simulink model "one_loop_dcmotor"  (R2022a)
settings: Solver=VariableStepAuto  StartTime=0.0  StopTime=10  MaxStep=1e-5  RelTol=1e-3
values from neighbouring files (symbols this model uses):
  Ce = 0.131    [params.m]
  Ra = 1.5    [params.m]
  TL = 0.0144    [params.m]
  Tm = 0.18    [params.m]
libraries: spsDCVoltageSourceLib x3, spsUniversalBridgeLib x3, simulink x3, spsVoltageMeasurementLib x3, spsMeanLib x2, spspowerguiLib x1
settings Model: Creator=lzd  LastModifiedBy=lzd

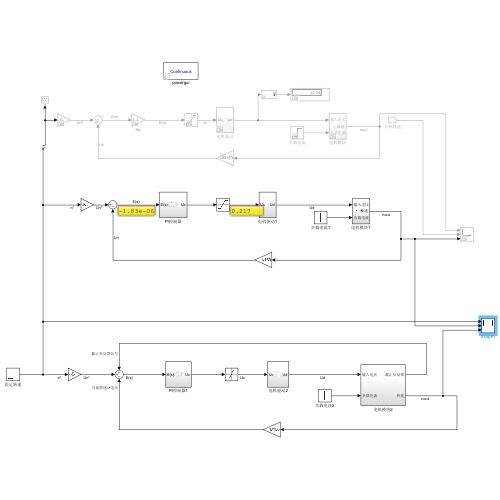
[thumbnail: Simulink's stored preview of the top-level diagram]
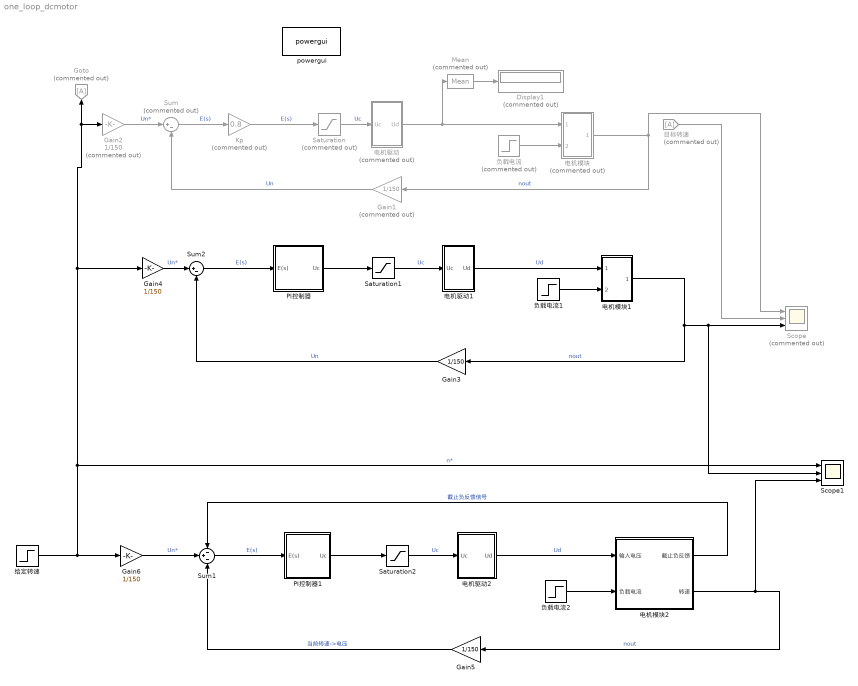
== system one_loop_dcmotor ==
  Display1 : Display  Commented=on
  Gain1 : Gain  Commented=on  Gain=1/150
  Gain2 : Gain  Commented=on  Gain=1/150
  Gain{3..6} (4 alike) : Gain  Gain=1/150
  Goto : Goto  Commented=on
  Kp : Gain  Commented=on  Gain=0.8
  Mean : spsMeanLib/Mean  Commented=on  Freq=60  Vinit=0  Ts=0
  PI控制器 : Subsystem
  PI控制器1 : Subsystem
  Saturation : Saturate  Commented=on  UpperLimit=5  LowerLimit=-5
  Saturation1 : Saturate  UpperLimit=5  LowerLimit=-5
  Saturation2 : Saturate  UpperLimit=5  LowerLimit=-5
  Scope : Scope  Commented=on  NumInputPorts=3
  Scope1 : Scope  NumInputPorts=3
  Sum : Sum  Commented=on  Inputs=|+-
  Sum1 : Sum  Inputs=-+-
  Sum2 : Sum  Inputs=|+-
  powergui : spspowerguiLib/powergui  Priority=1  SimulationMode=Continuous  SampleTime=50e-6  frequency=60  Iterations=50  frequencyindice=0  Pbase=100e6  ErrMax=1e-4  UnitsV=kV  UnitsW=MW  buscounter=0  FunctionMessages=off  echomessages=off  EnableUseOfTLC=off  CurrentSourceSwitches=off  DisableSnubberDevices=off  DisableRonSwitches=off  DisableVfSwitches=off  DisplayEquations=off  AutomaticDiscreteSolvers=off  SolverType=Tustin/Backward Euler (TBE)  Interpol=off  ExternalGateDelay=off  methode=off  Ts=100  x0status=blocks  SPID=on  SwTol=0  HookPort=off  NonlinearTolerance=1e-4  nMaxIteration=100  ContinueOnMaxIteration=off  RestoreLinks=warning  ResistiveCurrentMeasurement=off  Frange=[0:2:500]  Ylog=off  Xlog=on  ShowGrid=off  save=off  variable=ZData  structure=0  ZoomFFT=off  StartTime=0.0  cycles=1  DisplayStyle=1  fundamental=60  FreqAxis=off  MaxFrequency=1000  frequencyindicesteady=1  RmsSteady=1  display=off
  电机模块 : Subsystem  Commented=on
  电机模块1 : Subsystem
  电机模块2 : Subsystem
  电机驱动 : Subsystem  Commented=on
  电机驱动1 : Subsystem
  电机驱动2 : Subsystem
  目标转速 : From  Commented=on
  给定转速 : Step  Time=0.02  After=1300  SampleTime=0
  负载电流 : Step  Commented=on  Time=0.1  After=15.6  SampleTime=0
  负载电流1 : Step  Time=0.1  After=15.6  SampleTime=0
  负载电流2 : Step  Time=0.1  After=15.6  SampleTime=0
  wires:
  Mean/1 -> Display1/1
  电机模块/1(转速) -> Scope/1, Gain1/1  "nout"
  负载电流/1 -> 电机模块/2(负载电流)
  Sum/1 -> Kp/1  "E(s)"
  Gain1/1 -> Sum/2  "Un"
  Gain2/1 -> Sum/1  "Un*"
  电机驱动/1(Ud) -> 电机模块/1(输入电压), Mean/1
  Saturation/1 -> 电机驱动/1(Uc)  "Uc"
  目标转速/1 -> Scope/2
  Kp/1 -> Saturation/1  "E(s)"
  Saturation1/1 -> 电机驱动1/1(Uc)  "Uc"
  电机驱动1/1(Ud) -> 电机模块1/1(输入电压)  "Ud"
  Gain4/1 -> Sum2/1  "Un*"
  Gain3/1 -> Sum2/2  "Un"
  负载电流1/1 -> 电机模块1/2(负载电流)
  电机模块1/1(转速) -> Gain3/1, Scope1/2, Scope/3  "nout"
  Sum2/1 -> PI控制器/1(E(s))  "E(s)"
  PI控制器/1(Uc) -> Saturation1/1
  PI控制器1/1(Uc) -> Saturation2/1
  电机模块2/2(转速) -> Scope1/3, Gain5/1  "nout"
  负载电流2/1 -> 电机模块2/2(负载电流)
  给定转速/1 -> Scope1/1, Gain2/1, Goto/1, Gain4/1, Gain6/1  "n*"
  电机驱动2/1(Ud) -> 电机模块2/1(输入电压)  "Ud"
  Saturation2/1 -> 电机驱动2/1(Uc)  "Uc"
  Sum1/1 -> PI控制器1/1(E(s))  "E(s)"
  Gain6/1 -> Sum1/2  "Un*"
  电机模块2/1(截止负反馈) -> Sum1/1  "截止负反馈信号"
  Gain5/1 -> Sum1/3  "当前转速->电压"

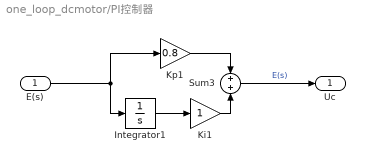
== system one_loop_dcmotor/PI控制器 ==
  E(s) : Inport
  Integrator1 : Integrator  LimitOutput=on  UpperSaturationLimit=5  LowerSaturationLimit=-5
  Ki1 : Gain
  Kp1 : Gain  Gain=0.8
  Sum3 : Sum  Inputs=+|+
  Uc : Outport
  wires:
  E(s)/1 -> Integrator1/1, Kp1/1
  Ki1/1 -> Sum3/2
  Integrator1/1 -> Ki1/1
  Kp1/1 -> Sum3/1
  Sum3/1 -> Uc/1  "E(s)"

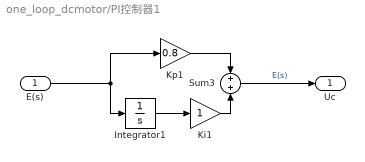
== system one_loop_dcmotor/PI控制器1 ==
  E(s) : Inport
  Integrator1 : Integrator  LimitOutput=on  UpperSaturationLimit=5  LowerSaturationLimit=-5
  Ki1 : Gain
  Kp1 : Gain  Gain=0.8
  Sum3 : Sum  Inputs=+|+
  Uc : Outport
  wires:
  Sum3/1 -> Uc/1  "E(s)"
  Kp1/1 -> Sum3/1
  Integrator1/1 -> Ki1/1
  Ki1/1 -> Sum3/2
  E(s)/1 -> Kp1/1, Integrator1/1

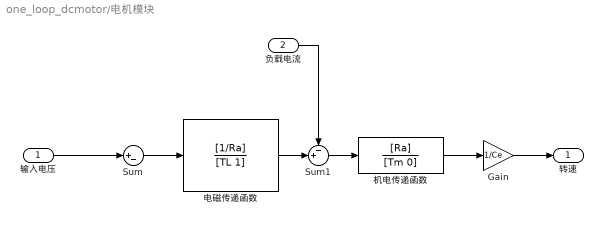
== system one_loop_dcmotor/电机模块 ==
  输入电压 : Inport
  负载电流 : Inport  Port=2
  Gain : Gain  Gain=1/Ce
  Sum : Sum  Inputs=|+-
  Sum1 : Sum  Inputs=-+|
  机电传递函数 : TransferFcn  Numerator=[Ra]  Denominator=[Tm 0]
  电磁传递函数 : TransferFcn  Numerator=[1/Ra]  Denominator=[TL 1]
  转速 : Outport
  wires:
  输入电压/1 -> Sum/1
  电磁传递函数/1 -> Sum1/2
  负载电流/1 -> Sum1/1
  Sum1/1 -> 机电传递函数/1
  机电传递函数/1 -> Gain/1
  Sum/1 -> 电磁传递函数/1
  Gain/1 -> 转速/1

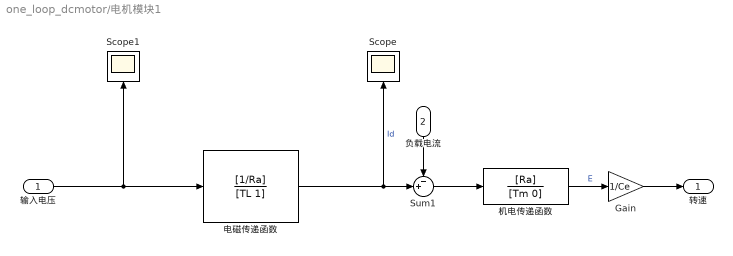
== system one_loop_dcmotor/电机模块1 ==
  输入电压 : Inport
  负载电流 : Inport  Port=2
  Gain : Gain  Gain=1/Ce
  Scope : Scope
  Scope1 : Scope
  Sum1 : Sum  Inputs=-+|
  机电传递函数 : TransferFcn  Numerator=[Ra]  Denominator=[Tm 0]
  电磁传递函数 : TransferFcn  Numerator=[1/Ra]  Denominator=[TL 1]
  转速 : Outport
  wires:
  Gain/1 -> 转速/1
  输入电压/1 -> 电磁传递函数/1, Scope1/1
  机电传递函数/1 -> Gain/1  "E"
  Sum1/1 -> 机电传递函数/1
  负载电流/1 -> Sum1/1
  电磁传递函数/1 -> Sum1/2, Scope/1  "Id"

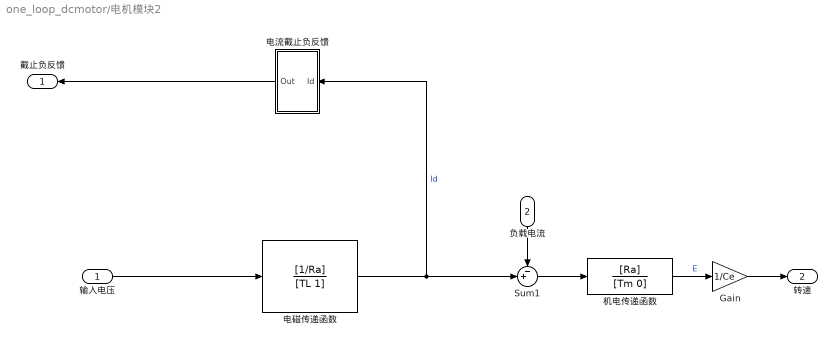
== system one_loop_dcmotor/电机模块2 ==
  输入电压 : Inport
  负载电流 : Inport  Port=2
  Gain : Gain  Gain=1/Ce
  Sum1 : Sum  Inputs=-+|
  机电传递函数 : TransferFcn  Numerator=[Ra]  Denominator=[Tm 0]
  电流截止负反馈 : Subsystem
  电磁传递函数 : TransferFcn  Numerator=[1/Ra]  Denominator=[TL 1]
  截止负反馈 : Outport
  转速 : Outport  Port=2
  wires:
  电磁传递函数/1 -> Sum1/2, 电流截止负反馈/1(Id)  "Id"
  负载电流/1 -> Sum1/1
  Sum1/1 -> 机电传递函数/1
  机电传递函数/1 -> Gain/1  "E"
  输入电压/1 -> 电磁传递函数/1
  Gain/1 -> 转速/1
  电流截止负反馈/1(Out) -> 截止负反馈/1

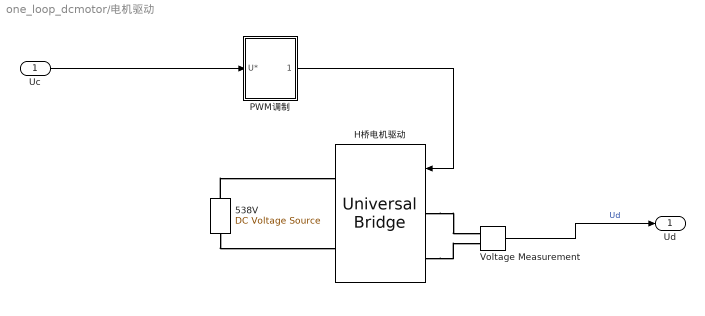
== system one_loop_dcmotor/电机驱动 ==
  Uc : Inport
  538V : spsDCVoltageSourceLib/DC Voltage Source  Amplitude=538  Measurements=None
  H桥电机驱动 : spsUniversalBridgeLib/Universal Bridge  Arms=2  SnubberResistance=1e5  SnubberCapacitance=inf  Device=MOSFET / Diodes  Ron=1e-3  Lon=0  ForwardVoltages="[  0  0  ]"  ForwardVoltage=0  GTOparameters=[ 10e-6 , 20e-6 ]  IGBTparameters=[ 1e-6 , 2e-6 ]  Measurements=None  Measurements_2=None  converterType=Rectifier
  PWM调制 : Subsystem
  Voltage Measurement : spsVoltageMeasurementLib/Voltage Measurement  PhasorSimulation=off  OutputType=Complex  PSBequivalent=0
  Ud : Outport
  wires:
  Voltage Measurement/1 -> Ud/1  "Ud"
  PWM调制/1(4*PWM) -> H桥电机驱动/1
  Uc/1 -> PWM调制/1(U*)
  connections:
  H桥电机驱动/LConn2 -- Voltage Measurement/LConn2
  538V/LConn1 -- H桥电机驱动/RConn2
  538V/RConn1 -- H桥电机驱动/RConn1
  H桥电机驱动/LConn1 -- Voltage Measurement/LConn1

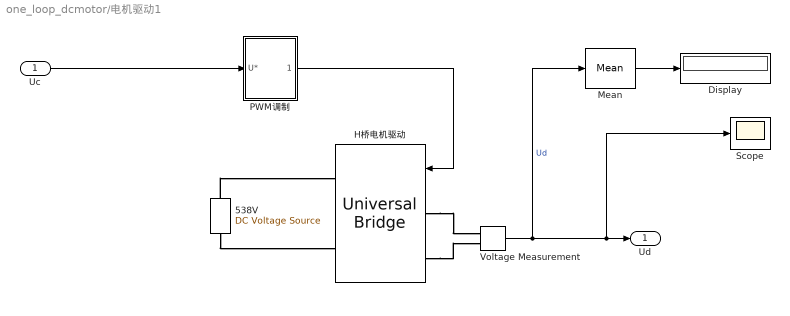
== system one_loop_dcmotor/电机驱动1 ==
  Uc : Inport
  538V : spsDCVoltageSourceLib/DC Voltage Source  Amplitude=538  Measurements=None
  Display : Display
  H桥电机驱动 : spsUniversalBridgeLib/Universal Bridge  Arms=2  SnubberResistance=1e5  SnubberCapacitance=inf  Device=MOSFET / Diodes  Ron=1e-3  Lon=0  ForwardVoltages="[  0  0  ]"  ForwardVoltage=0  GTOparameters=[ 10e-6 , 20e-6 ]  IGBTparameters=[ 1e-6 , 2e-6 ]  Measurements=None  Measurements_2=None  converterType=Rectifier
  Mean : spsMeanLib/Mean  Freq=50  Vinit=0  Ts=0
  PWM调制 : Subsystem
  Scope : Scope
  Voltage Measurement : spsVoltageMeasurementLib/Voltage Measurement  PhasorSimulation=off  OutputType=Complex  PSBequivalent=0
  Ud : Outport
  wires:
  Uc/1 -> PWM调制/1(U*)
  PWM调制/1(4*PWM) -> H桥电机驱动/1
  Voltage Measurement/1 -> Mean/1, Scope/1, Ud/1  "Ud"
  Mean/1 -> Display/1
  connections:
  H桥电机驱动/LConn1 -- Voltage Measurement/LConn1
  538V/RConn1 -- H桥电机驱动/RConn1
  538V/LConn1 -- H桥电机驱动/RConn2
  H桥电机驱动/LConn2 -- Voltage Measurement/LConn2

== system one_loop_dcmotor/电机驱动2 ==
  Uc : Inport
  538V : spsDCVoltageSourceLib/DC Voltage Source  Amplitude=538  Measurements=None
  H桥电机驱动 : spsUniversalBridgeLib/Universal Bridge  Arms=2  SnubberResistance=1e5  SnubberCapacitance=inf  Device=MOSFET / Diodes  Ron=1e-3  Lon=0  ForwardVoltages="[  0  0  ]"  ForwardVoltage=0  GTOparameters=[ 10e-6 , 20e-6 ]  IGBTparameters=[ 1e-6 , 2e-6 ]  Measurements=None  Measurements_2=None  converterType=Rectifier
  PWM调制 : Subsystem
  Voltage Measurement : spsVoltageMeasurementLib/Voltage Measurement  PhasorSimulation=off  OutputType=Complex  PSBequivalent=0
  Ud : Outport
  wires:
  Voltage Measurement/1 -> Ud/1  "Ud"
  PWM调制/1(4*PWM) -> H桥电机驱动/1
  Uc/1 -> PWM调制/1(U*)
  connections:
  H桥电机驱动/LConn2 -- Voltage Measurement/LConn2
  538V/LConn1 -- H桥电机驱动/RConn2
  538V/RConn1 -- H桥电机驱动/RConn1
  H桥电机驱动/LConn1 -- Voltage Measurement/LConn1

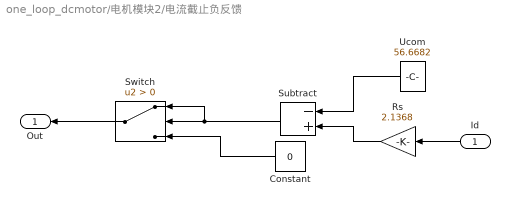
== system one_loop_dcmotor/电机模块2/电流截止负反馈 ==
  Id : Inport
  Constant : Constant  Value=0
  Rs : Gain  Gain=2.1368
  Subtract : Sum  Inputs=-+
  Switch : Switch  Criteria=u2 > Threshold  SaturateOnIntegerOverflow=off  InputSameDT=off
  Ucom : Constant  Value=56.6682
  Out : Outport
  wires:
  Subtract/1 -> Switch/2, Switch/1
  Id/1 -> Rs/1
  Rs/1 -> Subtract/2
  Constant/1 -> Switch/3
  Ucom/1 -> Subtract/1
  Switch/1 -> Out/1

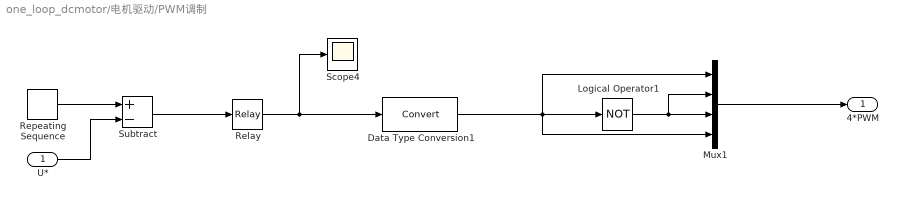
== system one_loop_dcmotor/电机驱动/PWM调制 ==
  U* : Inport
  Data Type Conversion1 : DataTypeConversion  SaturateOnIntegerOverflow=off  RndMeth=Floor
  Logical Operator1 : Logic  Operator=NOT  AllPortsSameDT=off  OutDataTypeStr=boolean
  Mux1 : Mux
  Relay : Relay  OnOutputValue=0  OffOutputValue=1
  Repeating Sequence : simulink/Sources/Repeating Sequence  rep_seq_t=[0 1/8000]  rep_seq_y=[-5 +5]
  Scope4 : Scope
  Subtract : Sum  Inputs=+-
  4*PWM : Outport
  wires:
  Relay/1 -> Scope4/1, Data Type Conversion1/1
  Data Type Conversion1/1 -> Mux1/4, Mux1/1, Logical Operator1/1
  Subtract/1 -> Relay/1
  Logical Operator1/1 -> Mux1/2, Mux1/3
  Repeating Sequence/1 -> Subtract/1
  Mux1/1 -> 4*PWM/1
  U*/1 -> Subtract/2

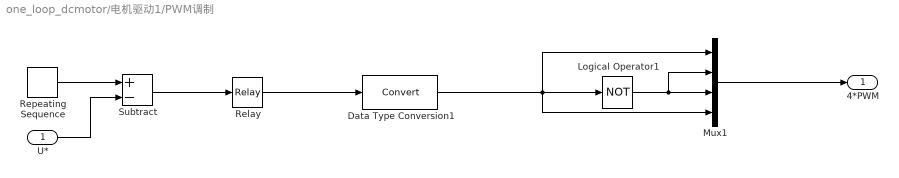
== system one_loop_dcmotor/电机驱动1/PWM调制 ==
  U* : Inport
  Data Type Conversion1 : DataTypeConversion  SaturateOnIntegerOverflow=off  RndMeth=Floor
  Logical Operator1 : Logic  Operator=NOT  AllPortsSameDT=off  OutDataTypeStr=boolean
  Mux1 : Mux
  Relay : Relay  OnOutputValue=0  OffOutputValue=1
  Repeating Sequence : simulink/Sources/Repeating Sequence  rep_seq_t=[0 1/8000]  rep_seq_y=[-5 +5]
  Subtract : Sum  Inputs=+-
  4*PWM : Outport
  wires:
  U*/1 -> Subtract/2
  Mux1/1 -> 4*PWM/1
  Repeating Sequence/1 -> Subtract/1
  Logical Operator1/1 -> Mux1/3, Mux1/2
  Subtract/1 -> Relay/1
  Data Type Conversion1/1 -> Logical Operator1/1, Mux1/1, Mux1/4
  Relay/1 -> Data Type Conversion1/1

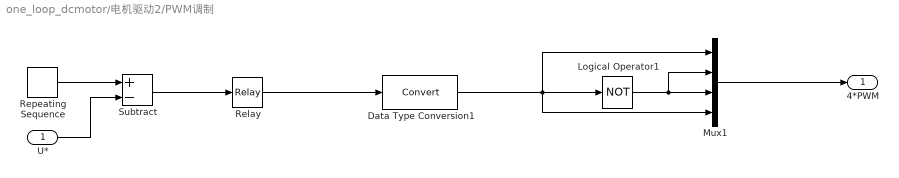
== system one_loop_dcmotor/电机驱动2/PWM调制 ==
  U* : Inport
  Data Type Conversion1 : DataTypeConversion  SaturateOnIntegerOverflow=off  RndMeth=Floor
  Logical Operator1 : Logic  Operator=NOT  AllPortsSameDT=off  OutDataTypeStr=boolean
  Mux1 : Mux
  Relay : Relay  OnOutputValue=0  OffOutputValue=1
  Repeating Sequence : simulink/Sources/Repeating Sequence  rep_seq_t=[0 1/8000]  rep_seq_y=[-5 +5]
  Subtract : Sum  Inputs=+-
  4*PWM : Outport
  wires:
  Relay/1 -> Data Type Conversion1/1
  Data Type Conversion1/1 -> Mux1/4, Mux1/1, Logical Operator1/1
  Subtract/1 -> Relay/1
  Logical Operator1/1 -> Mux1/2, Mux1/3
  Repeating Sequence/1 -> Subtract/1
  Mux1/1 -> 4*PWM/1
  U*/1 -> Subtract/2
